simulink model "Modelo_con_sweep_ctes_variables_obs"  (R2020a)
settings: Solver=ode15s  StartTime=0.0  StopTime=10  FixedStep=0.001  MaxStep=0.0001  RelTol=1e-3
undefined symbols (not defined in the file): A, A_reduc, Amp, B, B_reduc, Bdlol, C_reduc, Cc, D, f, f0, I_max, K_motor_virtual, L, Li, Lobs, R, R_control, v0, x0, ZOH
libraries: dspstat3 x1
settings Model: Creator=Noxi-PC  LastModifiedBy=Noxi-PC

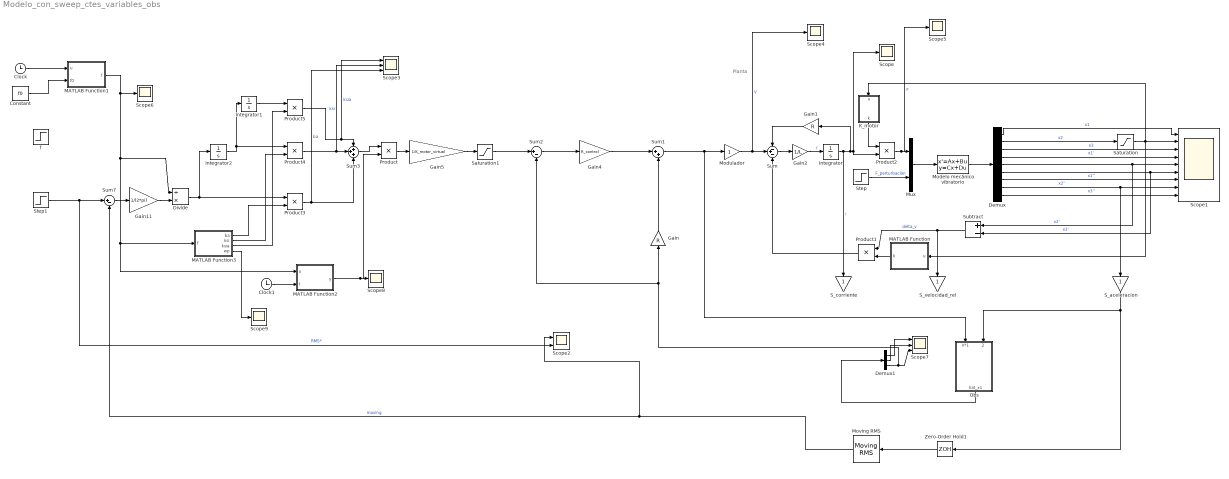
== system Modelo_con_sweep_ctes_variables_obs ==
  note: Planta
  Clock : Clock
  Clock1 : Clock
  Constant : Constant  Value=f0
  Demux : Demux  Outputs=9
  Demux1 : Demux  Outputs=3
  Divide : Product  Inputs=/*
  Gain : Gain  Gain=R
  Gain1 : Gain  Gain=R
  Gain11 : Gain  Gain=1/(2*pi)
  Gain2 : Gain  Gain=1/L
  Gain4 : Gain  Gain=R_control
  Gain5 : Gain  Gain=1/K_motor_virtual
  Integrator : Integrator
  Integrator1 : Integrator
  Integrator2 : Integrator
  K_motor : MATLAB Function  TreatAsAtomicUnit=on
  MATLAB Function : MATLAB Function  TreatAsAtomicUnit=on
  MATLAB Function1 : MATLAB Function  TreatAsAtomicUnit=on
  MATLAB Function2 : MATLAB Function  TreatAsAtomicUnit=on
  MATLAB Function3 : MATLAB Function  TreatAsAtomicUnit=on
  Modelo mecánico vibratorio : StateSpace  A=A  B=B  C=Cc  D=D  InitialCondition=[x0,v0]
  Modulador : Gain
  Moving RMS : dspstat3/Moving RMS  Method=Sliding window  ForgettingFactorPort=off  SpecifyWindowLength=on  WindowLength=Ventana  ForgettingFactor=0.99  SimulateUsing=Code generation
      settings: SourceProductBaseCode=DS
  Mux : Mux  Inputs=2
  Obs : Subsystem
  Product{,1..5} (6 alike) : Product
  S_aceleracion : Gain
  S_corriente : Gain
  S_velocidad_rel : Gain
  Saturation : Saturate  UpperLimit=12.7e-3  LowerLimit=-12.7e-3
  Saturation1 : Saturate  UpperLimit=I_max  LowerLimit=-I_max
  Scope{,4..6,8..9} (6 alike) : Scope
  Scope1 : Scope  NumInputPorts=9
  Scope2 : Scope  NumInputPorts=2
  Scope3 : Scope  NumInputPorts=3
  Scope7 : Scope  NumInputPorts=3
  Step : Step  Time=3  After=0  SampleTime=0
  Step1 : Step  After=Amp/sqrt(2)  SampleTime=0
  Subtract : Sum  Inputs=+-
  Sum : Sum  Inputs=-+-
  Sum1 : Sum  Inputs=|++
  Sum2 : Sum  Inputs=|+-
  Sum3 : Sum  Inputs=+++
  Sum7 : Sum  Inputs=|+-
  Zero-Order Hold1 : ZeroOrderHold  SampleTime=ZOH
  f : Step  Time=0  After=f  SampleTime=0
  wires:
  Modelo mecánico vibratorio/1 -> Demux/1
  Demux/1 -> Scope1/1  "x1"
  Demux/2 -> Saturation/1  "x2"
  Demux/3 -> Scope1/3  "x3"
  Demux/4 -> Scope1/4  "x1'"
  Demux/5 -> Scope1/5, Subtract/1  "x2'"
  Demux/6 -> Scope1/6, Subtract/2  "x3'"
  Demux/7 -> Scope1/7  "x1''"
  Demux/8 -> Scope1/8, S_aceleracion/1  "x2''"
  Demux/9 -> Scope1/9  "x3''"
  Mux/1 -> Modelo mecánico vibratorio/1
  Sum/1 -> Gain2/1
  Integrator/1 -> S_corriente/1, Product2/2, Scope/1, Gain1/1  "i"
  Gain1/1 -> Sum/1
  Gain2/1 -> Integrator/1  "i'"
  Step/1 -> Mux/2  "F_perturbación"
  Product1/1 -> Sum/3
  Subtract/1 -> Product1/1, S_velocidad_rel/1  "delta_v"
  Modulador/1 -> Scope4/1, Sum/2  "V"
  Sum2/1 -> Gain4/1
  Gain5/1 -> Saturation1/1
  Gain4/1 -> Sum1/1
  Product4/1 -> Sum3/2, Scope3/2  "ksi"
  Product3/1 -> Sum3/3, Scope3/3  "ba"
  Integrator2/1 -> Product4/1, Integrator1/1
  S_aceleracion/1 -> Obs/2(acc_medida1), Zero-Order Hold1/1
  Zero-Order Hold1/1 -> Moving RMS/1
  Step1/1 -> Scope2/2, Sum7/1  "RMS*"
  Moving RMS/1 -> Scope2/1, Sum7/2  "moving"
  Sum7/1 -> Gain11/1
  Sum3/1 -> Product/1
  Saturation/1 -> K_motor/1(u), MATLAB Function/1(u), Scope1/2
  Product2/1 -> Scope5/1, Mux/1  "F"
  K_motor/1(k) -> Product2/1
  MATLAB Function/1(k) -> Product1/2
  Sum1/1 -> Obs/1(V*1), Modulador/1
  Divide/1 -> Product3/1, Integrator2/1
  Gain11/1 -> Divide/2
  Product/1 -> Gain5/1
  Saturation1/1 -> Sum2/1
  Clock/1 -> MATLAB Function1/1(u)
  MATLAB Function1/1(f) -> Divide/1, MATLAB Function3/1(f), MATLAB Function2/1(u), Scope6/1
  Clock1/1 -> MATLAB Function2/2(t)
  MATLAB Function2/1(y) -> Product/2, Scope8/1
  MATLAB Function3/1(ba) -> Product3/2
  MATLAB Function3/2(ksi) -> Product4/2
  Integrator1/1 -> Product5/1
  MATLAB Function3/3(ksia) -> Product5/2
  MATLAB Function3/4(wp) -> Scope9/1
  Constant/1 -> MATLAB Function1/2(f0)
  Gain/1 -> Sum1/2
  Product5/1 -> Scope3/1, Sum3/1  "ksia"
  Obs/1(hat_x1) -> Demux1/1
  Demux1/1 -> Scope7/1
  Demux1/2 -> Scope7/2
  Demux1/3 -> Sum2/2, Gain/1, Scope7/3

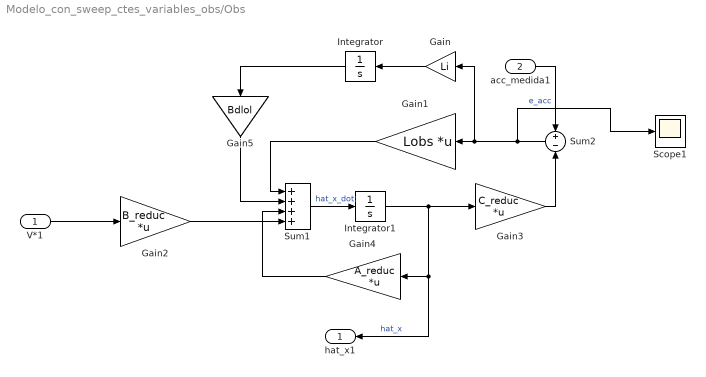
== system Modelo_con_sweep_ctes_variables_obs/Obs ==
  V*1 : Inport
  acc_medida1 : Inport  Port=2
  Gain : Gain  Gain=Li
  Gain1 : Gain  Gain=Lobs  Multiplication=Matrix(K*u)
  Gain2 : Gain  Gain=B_reduc  Multiplication=Matrix(K*u)
  Gain3 : Gain  Gain=C_reduc  Multiplication=Matrix(K*u)
  Gain4 : Gain  Gain=A_reduc  Multiplication=Matrix(K*u)
  Gain5 : Gain  Gain=Bdlol
  Integrator : Integrator
  Integrator1 : Integrator
  Scope1 : Scope
  Sum1 : Sum  Inputs=++++
  Sum2 : Sum  Inputs=+|-
  hat_x1 : Outport  VectorParamsAs1DForOutWhenUnconnected=off
  wires:
  Gain1/1 -> Sum1/1
  Gain4/1 -> Sum1/3
  V*1/1 -> Gain2/1
  Sum2/1 -> Scope1/1, Gain/1, Gain1/1  "e_acc"
  Integrator1/1 -> hat_x1/1, Gain4/1, Gain3/1  "hat_x"
  Sum1/1 -> Integrator1/1  "hat_x_dot"
  acc_medida1/1 -> Sum2/1
  Gain3/1 -> Sum2/2
  Gain/1 -> Integrator/1
  Integrator/1 -> Gain5/1
  Gain5/1 -> Sum1/2
  Gain2/1 -> Sum1/4

== matlab function Modelo_con_sweep_ctes_variables_obs/K_motor ==
  data: u input; k output
function k = fcn(u)
coefs = [1.88388325014986e-06,1.21220914940963e-07,-0.000604988778285308,-0.000369001905871298,-0.0433714523559467,-0.0474444922489168,51.4222931299995];

k = coefs(1)*u^6+coefs(2)*u^5+coefs(3)*u^4+coefs(4)*u^3+coefs(5)*u^2+coefs(6)*u^1+coefs(7);

== matlab function Modelo_con_sweep_ctes_variables_obs/MATLAB Function ==
  data: u input; k output
function k= fcn(u)
coefs = [1.88388325014986e-06,1.21220914940963e-07,-0.000604988778285308,-0.000369001905871298,-0.0433714523559467,-0.0474444922489168,51.4222931299995];

k = coefs(1)*u^6+coefs(2)*u^5+coefs(3)*u^4+coefs(4)*u^3+coefs(5)*u^2+coefs(6)*u^1+coefs(7);

== matlab function Modelo_con_sweep_ctes_variables_obs/MATLAB Function1 ==
  data: u input; f output; f0 input
function f = fcn(u,f0)

f = f0* 2^(2*u/60);

== matlab function Modelo_con_sweep_ctes_variables_obs/MATLAB Function2 ==
  data: u input; y output; t input
function y = fcn(u,t)

y = sin(2*pi*u*t);

== matlab function Modelo_con_sweep_ctes_variables_obs/MATLAB Function3 ==
  data: f input; ba output; ksi output; ksia output; wp output
function [ba,ksi,ksia,wp] = fcn(f)
m_movil = 0.94;
zita = 0.7;
wp = wpfreq(f);
ba = m_movil*(2*zita+1)*wp;
ksi = m_movil*(2*zita+1)*wp^2*10;
ksia = m_movil*wp^3;
end

function wp = wpfreq(f)
    % Tabla de frecuencia (Hz) y valores correspondientes de wp
    freq_table = [ ...
          5,  10,  20,  25,  30,  40,  50,  60,  70,  80, ...
         90, 100, 200, 300, 400, 500, 600,700,739,800, 853, 1000, 1134,1200, 1300, 1450, 1500, 2000];

    wp_table = [ ...
         20,  10,  10,  20,  22,  25,  25,  25,  30,  30, ...
         40,  40,  50,  50,  70, 120,120,120, 250, 120, 200,  200, 150,150, 200, 200,  120,  200];

    % Interpolación lineal
    wp = interp1(freq_table, wp_table, f, 'linear', 'extrap');
end
